simulink model "ModDemodAMDSB"  (Simulink 7.5)
settings: Solver=ode45  StartTime=0.0  StopTime=10.0  RelTol=1e-3
settings Model: Creator=ele10168  LastModifiedBy=ele10168

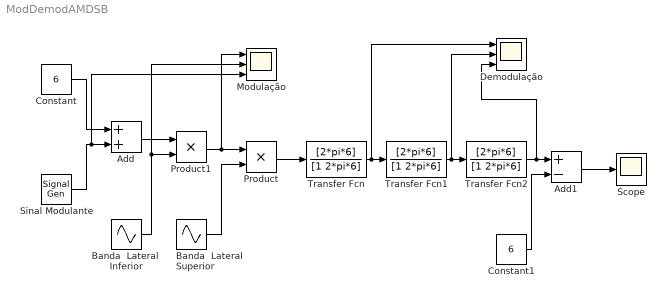
== system ModDemodAMDSB ==
  Add : Sum  OutDataType=fixdt(1, 16)  OutScaling=2^-10  SampleTime=0.001
  Add1 : Sum  Inputs=+-  OutDataType=fixdt(1, 16)  OutScaling=2^-10  SampleTime=0.001
  Banda  Lateral  Inferior : Sin  Amplitude=1  Bias=0  Frequency=2*pi*20  Phase=pi/2  Samples=10  SampleTime=0.001  Offset=0
  Banda  Lateral  Superior : Sin  Amplitude=2  Bias=0  Frequency=2*pi*20  Phase=pi/2  Samples=10  SampleTime=0.001  Offset=0
  Constant : Constant  Value=6  OutDataType=fixdt(1, 16)  OutScaling=2^0  SampleTime=0.001
  Constant1 : Constant  Value=6  OutDataType=fixdt(1, 16)  OutScaling=2^0  SampleTime=0.001
  Demodulação : Scope  NumInputPorts=3
      settings: YMin=-5~-5~-5  YMax=5~5~5
  Modulação : Scope  NumInputPorts=3
      settings: YMin=-5~-5~-5  YMax=5~5~5  SaveName=ScopeData2
  Product : Product  OutDataType=fixdt(1, 16)  OutScaling=2^0  SampleTime=0.001  RndMeth=Zero
  Product1 : Product  OutDataType=fixdt(1, 16)  OutScaling=2^0  SampleTime=0.001  RndMeth=Zero
  Scope : Scope
  Sinal Modulante : SignalGenerator  Amplitude=3
  Transfer Fcn : TransferFcn  Numerator=[2*pi*6]  Denominator=[1 2*pi*6]
  Transfer Fcn1 : TransferFcn  Numerator=[2*pi*6]  Denominator=[1 2*pi*6]
  Transfer Fcn2 : TransferFcn  Numerator=[2*pi*6]  Denominator=[1 2*pi*6]
  wires:
  Constant/1 -> Add/1
  Sinal Modulante/1 -> Add/2, Modulação/3
  Banda  Lateral  Inferior/1 -> Product1/2, Modulação/2
  Add/1 -> Product1/1
  Product1/1 -> Product/1, Modulação/1
  Banda  Lateral  Superior/1 -> Product/2
  Product/1 -> Transfer Fcn/1
  Transfer Fcn/1 -> Transfer Fcn1/1, Demodulação/1
  Transfer Fcn1/1 -> Transfer Fcn2/1, Demodulação/2
  Transfer Fcn2/1 -> Add1/1, Demodulação/3
  Constant1/1 -> Add1/2
  Add1/1 -> Scope/1
